simulink model "simulink_hils"  (R2026a)
settings: Solver=VariableStepAuto  StopTime=30
undefined symbols (not defined in the file or in its folder): egoVehicle, scenarioConfig
libraries: drivingscenarioandsensors x5, sim3dautolib x3, sim3dlib x1
settings Model: Creator=johnny  LastModifiedBy=johnny

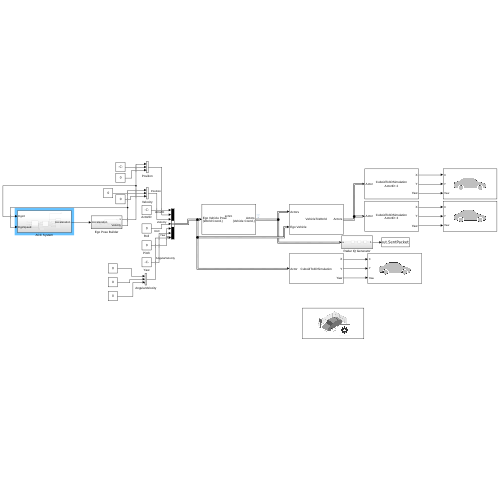
[thumbnail: Simulink's stored preview of the top-level diagram]
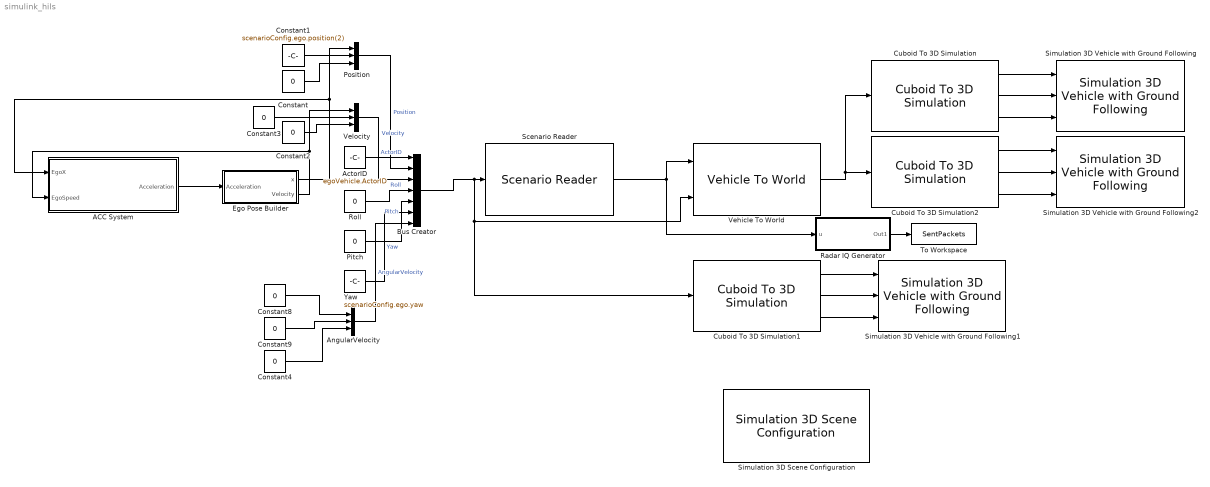
== system simulink_hils ==
  ACC System : Subsystem
  ActorID : Constant  Value=egoVehicle.ActorID
  AngularVelocity : Concatenate  NumInputs=3  Mode=Multidimensional array  ConcatenateDimension=2
  Bus Creator : BusCreator  Inputs=7  OutDataTypeStr=Bus: EgoPoseBus  NonVirtualBus=on
  Constant{,2..4,8..9} (6 alike) : Constant  Value=0
  Constant1 : Constant  Value=scenarioConfig.ego.position(2)
  Cuboid To 3D Simulation : drivingscenarioandsensors/Cuboid To 3D Simulation  SpecifyActorID=on  ActorIDToConvert=2  SimulateUsing=Interpreted execution
  Cuboid To 3D Simulation1 : drivingscenarioandsensors/Cuboid To 3D Simulation  SpecifyActorID=off  ActorIDToConvert=1  SimulateUsing=Interpreted execution
  Cuboid To 3D Simulation2 : drivingscenarioandsensors/Cuboid To 3D Simulation  SpecifyActorID=on  ActorIDToConvert=3  SimulateUsing=Interpreted execution
  Ego Pose Builder : Subsystem
  Pitch : Constant  Value=0
  Position : Concatenate  NumInputs=3  Mode=Multidimensional array  ConcatenateDimension=2
  Radar IQ Generator : Subsystem
  Roll : Constant  Value=0
  Scenario Reader : drivingscenarioandsensors/Scenario Reader  ScenarioSource=From workspace  ScenarioFileName=EgoVehicleGoesStraight.mat  ScenarioVariableName=scnro  OutputCoordinateSystem=Vehicle coordinates  EgoVehicleSource=Input port  EgoVehicleActorID=1  OrientVehiclesOnRoad=off  OutputEgoVehiclePose=on  OutputEgoVehicleState=off  SampleTime=0.01  LaneBoundaryOutput=None  LaneBoundaryDistance=0:0.5:9.5  LaneBoundaryLocation=Center of lane markings  BusNameSource=Auto  BusName=BusActors  BusNumActorsSource=Property  BusNumActors=8  BusName2Source=Auto  BusName2=BusLaneBoundaries  BusNumLaneBoundariesSource=Scenario  BusNumLaneBoundaries=10  BusName3Source=Auto  BusName3=BusEgoActor  BusName4Source=Auto  BusName4=BusEgoState  ShowCoordinateLabels=on  SimulateUsing=Interpreted execution
  Simulation 3D Scene Configuration : sim3dlib/Simulation 3D Scene Configuration  Priority=0  ProjectFormat=Default Scenes  SceneDesc=Straight road  ProjectName=/usr/local/MATLAB/R2026a/toolbox/shared/sim3d_projects/automotive_project_linux/UE/LinuxNoEditor/VehicleSimulation.sh  ScenePath=/Game/Maps/HwStrght  EnableOpenDRIVE=off  vehTagList={'Custom';'Scene Origin';'SimulinkVehicle1';'SimulinkVehicle2';'TargetVehicle'}  vehTag=SimulinkVehicle1  AttachedCameraRelativeTranslation=[0 0 0]  FreeCameraDefaultInitialTranslation=[-6, 0, 2]  AttachedCameraRelativeRotation=[0, -15, 0]  FreeCameraDefaultInitialRotation=[0, -15, 0]  ViewpointName=Custom  FreeCameraInitialTranslation=[0, 0, 0]  FreeCameraInitialRotation=[0, 0, 0]  OpVisEn=off  Ts=.02  EnableWindow=on  EnableRemoteAccess=off  SimulationMode=CoSimulation  SimulateUsing=Interpreted execution  EnableAnimationRecording=off  OverrideDefaultRecording=off  AnimationRecordingFileName=sim3dAnimation.mat  AnimationRecordingInterval=[0 inf]  EnableWeather=off  SunAzimuth=90  SunAltitude=40.0  EnableGeospatialSun=off  Latitude=0  Longitude=0  Date=2023-01-01  Time=10:30:00  GeoTimeZone=-5.0  SunDaylightSaving=off  wind=1  clouds=10  EnableVolumetricClouds=off  CloudCoverage=0  CloudAltitude=6  fog=0  rain=0  RaindropsEffect=off  SnowDensity=0  EnableGeospatial=off  TilesetSource=Earth terrain  UseTrueOrigin=off  OriginHeight=200  OriginLatitude=40.744652  OriginLongitude=-73.988864  MapStyle=Aerial  AdditionalAssetIDs=[]  UseAdvancedSunSky=off  SolarTime=11  TimeZone=-5  Day=21  Month=9  Year=2022  UseDaylightSavingTime=on  DSTStartDay=10  DSTStartMonth=3  DSTEndDay=3  DSTEndMonth=11  DSTSwitchHour=2  sensorTag=MainCamera1  sensorId=1  sensorName=MainCamera1  mountLoc=Origin  offsetFlag=off  tmountOffset=[0, 0, 0]  rmountOffset=[0, 0, 0]  HorizontalResolution=1280  VerticalResolution=720  HorizontalFOV=60  mountPoint=[0 0 0]  mountOrientation=[0 0 0]  aMode=5  ID=1  GeoTrigger=Inactive  ViewNameList={'Custom'}  ViewTranslationList={'[0 0 0]'}  ViewRotationList={'[0 0 0]'}
      settings: LibrarySourceBlock=sl3dlib/Simulation 3D/Environment/Simulation 3D Scene Configuration
  Simulation 3D Vehicle with Ground Following : sim3dautolib/Simulation 3D Vehicle with Ground Following  Priority=-1  PassVehMesh=Muscle car  MeshPath=/MathWorksAutomotiveContent/Vehicles/Muscle/Meshes/SK_MuscleCar.SK_MuscleCar  TrackWidth=1.9  WheelBase=3  WheelRadius=0.35  VehColor=Blue  CoordinateSystem=ISO8855  InitialPos=[0, 0, 0]  InitialRot=[0, 0, 0]  ActorName=TargetVehicle  SampleTime=-1  ActorType=SimulinkVehicle  ID=C  aMode=3  ActorTag=TargetVehicle  CoordinateScheme=0  VehLightsControl=off  HeadlightColor=[ 1, 1, 1 ]  HighBeamIntensity=100000  LowBeamIntensity=60000  HighBeamConeAngle=70  LowBeamConeAngle=70  LeftHeadlightOrientation=[ 0, 0 ]  RightHeadlightOrientation=[ 0, 0 ]  BrakelightIntensity=500  ReverselightIntensity=500  SignallightIntensity=500  SignallightPeriod=1  SignalPulseWidth=50  TransformOutportEnabled=off
      settings: LibrarySourceBlock=drivingsim3d/Simulation 3D Vehicle with Ground Following
  Simulation 3D Vehicle with Ground Following1 : sim3dautolib/Simulation 3D Vehicle with Ground Following  Priority=-1  PassVehMesh=Muscle car  MeshPath=/MathWorksAutomotiveContent/Vehicles/Muscle/Meshes/SK_MuscleCar.SK_MuscleCar  TrackWidth=1.9  WheelBase=3  WheelRadius=0.35  VehColor=Red  CoordinateSystem=ISO8855  InitialPos=[0, 0, 0]  InitialRot=[0, 0, 0]  ActorName=SimulinkVehicle1  SampleTime=-1  ActorType=SimulinkVehicle  ID=1  aMode=3  ActorTag=SimulinkVehicle1  CoordinateScheme=0  VehLightsControl=off  HeadlightColor=[ 1, 1, 1 ]  HighBeamIntensity=100000  LowBeamIntensity=60000  HighBeamConeAngle=70  LowBeamConeAngle=70  LeftHeadlightOrientation=[ 0, 0 ]  RightHeadlightOrientation=[ 0, 0 ]  BrakelightIntensity=500  ReverselightIntensity=500  SignallightIntensity=500  SignallightPeriod=1  SignalPulseWidth=50  TransformOutportEnabled=off
      settings: LibrarySourceBlock=drivingsim3d/Simulation 3D Vehicle with Ground Following
  Simulation 3D Vehicle with Ground Following2 : sim3dautolib/Simulation 3D Vehicle with Ground Following  Priority=-1  PassVehMesh=Muscle car  MeshPath=/MathWorksAutomotiveContent/Vehicles/Muscle/Meshes/SK_MuscleCar.SK_MuscleCar  TrackWidth=1.9  WheelBase=3  WheelRadius=0.35  VehColor=Red  CoordinateSystem=ISO8855  InitialPos=[0, 0, 0]  InitialRot=[0, 0, 0]  ActorName=SimulinkVehicle2  SampleTime=-1  ActorType=SimulinkVehicle  ID=2  aMode=3  ActorTag=SimulinkVehicle2  CoordinateScheme=0  VehLightsControl=off  HeadlightColor=[ 1, 1, 1 ]  HighBeamIntensity=100000  LowBeamIntensity=60000  HighBeamConeAngle=70  LowBeamConeAngle=70  LeftHeadlightOrientation=[ 0, 0 ]  RightHeadlightOrientation=[ 0, 0 ]  BrakelightIntensity=500  ReverselightIntensity=500  SignallightIntensity=500  SignallightPeriod=1  SignalPulseWidth=50  TransformOutportEnabled=off
      settings: LibrarySourceBlock=drivingsim3d/Simulation 3D Vehicle with Ground Following
  To Workspace : ToWorkspace  VariableName=SentPackets  SaveFormat=Timeseries  SampleTime=-1
  Vehicle To World : drivingscenarioandsensors/Vehicle To World  BusNameSource=Auto  BusName=BusVehicleToWorldActors  SimulateUsing=Interpreted execution
  Velocity : Concatenate  NumInputs=3  Mode=Multidimensional array  ConcatenateDimension=2
  Yaw : Constant  Value=scenarioConfig.ego.yaw
  wires:
  Scenario Reader/1 -> Vehicle To World/1, Radar IQ Generator/1(u)
  Cuboid To 3D Simulation/1 -> Simulation 3D Vehicle with Ground Following/1
  Cuboid To 3D Simulation/2 -> Simulation 3D Vehicle with Ground Following/2
  Cuboid To 3D Simulation/3 -> Simulation 3D Vehicle with Ground Following/3
  Cuboid To 3D Simulation1/1 -> Simulation 3D Vehicle with Ground Following1/1
  Cuboid To 3D Simulation1/2 -> Simulation 3D Vehicle with Ground Following1/2
  Cuboid To 3D Simulation1/3 -> Simulation 3D Vehicle with Ground Following1/3
  Ego Pose Builder/1(x) -> Position/1, ACC System/1(EgoX)
  Constant/1 -> Position/3
  Constant1/1 -> Position/2
  Constant2/1 -> Velocity/3
  Constant3/1 -> Velocity/2
  Ego Pose Builder/2(Velocity) -> Velocity/1, ACC System/2(EgoSpeed)
  Constant8/1 -> AngularVelocity/1
  Constant9/1 -> AngularVelocity/2
  Constant4/1 -> AngularVelocity/3
  ActorID/1 -> Bus Creator/1  "ActorID"
  Position/1 -> Bus Creator/2  "Position"
  Velocity/1 -> Bus Creator/3  "Velocity"
  Roll/1 -> Bus Creator/4  "Roll"
  Pitch/1 -> Bus Creator/5  "Pitch"
  Yaw/1 -> Bus Creator/6  "Yaw"
  AngularVelocity/1 -> Bus Creator/7  "AngularVelocity"
  Bus Creator/1 -> Vehicle To World/2, Cuboid To 3D Simulation1/1, Scenario Reader/1
  Vehicle To World/1 -> Cuboid To 3D Simulation2/1, Cuboid To 3D Simulation/1
  Radar IQ Generator/1(Out1) -> To Workspace/1
  Cuboid To 3D Simulation2/3 -> Simulation 3D Vehicle with Ground Following2/3
  Cuboid To 3D Simulation2/2 -> Simulation 3D Vehicle with Ground Following2/2
  Cuboid To 3D Simulation2/1 -> Simulation 3D Vehicle with Ground Following2/1
  ACC System/1(Acceleration) -> Ego Pose Builder/1(Acceleration)

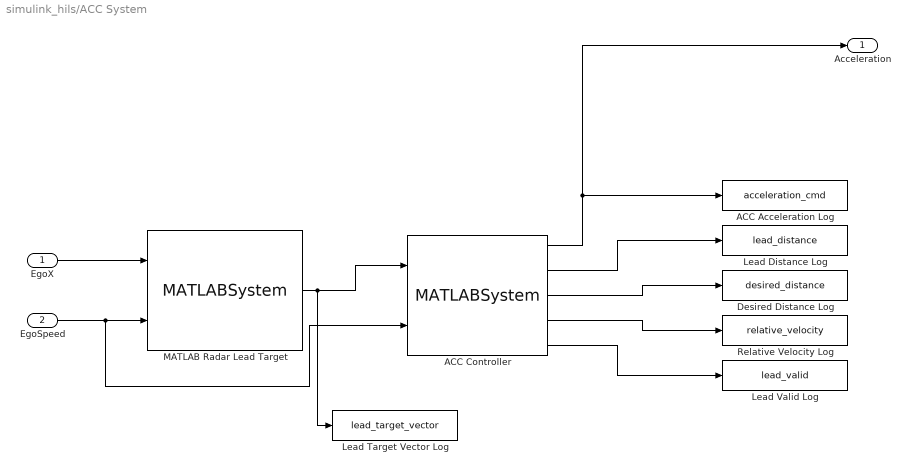
== system simulink_hils/ACC System ==
  EgoX : Inport
  EgoSpeed : Inport  Port=2
  ACC Acceleration Log : ToWorkspace  VariableName=acceleration_cmd  SaveFormat=Timeseries  SampleTime=-1
  ACC Controller : MATLABSystem  System=ACCControllerVector  SetSpeed=20.0  MinDistance=10.0  TimeHeadway=1.0  KpSpeed=2.5  KpGap=1.2  KvRelative=2.5  MaxAcceleration=4.0  MaxDeceleration=-10.0  SampleTime=0.01  SimulateUsing=Interpreted execution
      mask Type: ACCControllerVector
  Desired Distance Log : ToWorkspace  VariableName=desired_distance  SaveFormat=Timeseries  SampleTime=-1
  Lead Distance Log : ToWorkspace  VariableName=lead_distance  SaveFormat=Timeseries  SampleTime=-1
  Lead Target Vector Log : ToWorkspace  VariableName=lead_target_vector  SaveFormat=Timeseries  SampleTime=-1
  Lead Valid Log : ToWorkspace  VariableName=lead_valid  SaveFormat=Timeseries  SampleTime=-1
  MATLAB Radar Lead Target : MATLABSystem  System=MatlabRadarLeadTargetVectorSource  LaneHalfWidth=1.8  SampleTime=0.1  SimulateUsing=Interpreted execution
      mask Type: MatlabRadarLeadTargetVectorSource
  Relative Velocity Log : ToWorkspace  VariableName=relative_velocity  SaveFormat=Timeseries  SampleTime=-1
  Acceleration : Outport
  wires:
  EgoX/1 -> MATLAB Radar Lead Target/1
  EgoSpeed/1 -> ACC Controller/2, MATLAB Radar Lead Target/2
  MATLAB Radar Lead Target/1 -> ACC Controller/1, Lead Target Vector Log/1
  ACC Controller/1 -> Acceleration/1, ACC Acceleration Log/1
  ACC Controller/2 -> Lead Distance Log/1
  ACC Controller/3 -> Desired Distance Log/1
  ACC Controller/4 -> Relative Velocity Log/1
  ACC Controller/5 -> Lead Valid Log/1

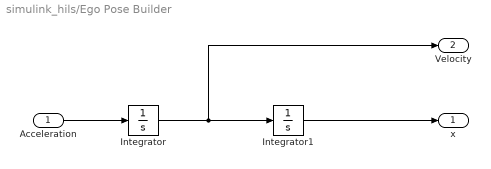
== system simulink_hils/Ego Pose Builder ==
  Acceleration : Inport
  Integrator : Integrator  InitialCondition=scenarioConfig.ego.initialSpeed
  Integrator1 : Integrator  InitialCondition=scenarioConfig.ego.position(1)
  x : Outport
  Velocity : Outport  Port=2
  wires:
  Acceleration/1 -> Integrator/1
  Integrator/1 -> Velocity/1, Integrator1/1
  Integrator1/1 -> x/1

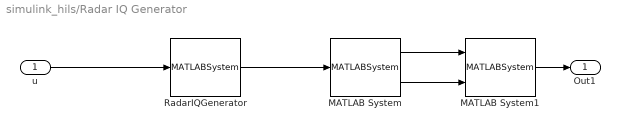
== system simulink_hils/Radar IQ Generator ==
  u : Inport
  MATLAB System : MATLABSystem  System=RadarPacketizer  SimulateUsing=Interpreted execution
      mask Type: RadarPacketizer
  MATLAB System1 : MATLABSystem  System=RadarUdpSender  DestinationIP=10.0.0.3  DestinationPort=5000  SimulateUsing=Interpreted execution
      mask Type: RadarUdpSender
  RadarIQGenerator : MATLABSystem  System=RadarIQGenerator  SimulateUsing=Interpreted execution
      mask Type: RadarIQGenerator
  Out1 : Outport
  wires:
  u/1 -> RadarIQGenerator/1
  RadarIQGenerator/1 -> MATLAB System/1
  MATLAB System/2 -> MATLAB System1/2
  MATLAB System/1 -> MATLAB System1/1
  MATLAB System1/1 -> Out1/1
